simulink model "Octocopter2D_04StatesLin"  (R2020b)
settings: Solver=VariableStepAuto  StartTime=0.0  StopTime=20  RelTol=1e-3
undefined symbols (not defined in the file): A, ACmp, B1, B2, BCmp, C2, CCmp, D21, DCmp, K, xInit
settings Model: Creator=jeremie  LastModifiedBy=jeremie
settings DebuggingCC: ArithmeticOperatorsInVariantConditions=warning
settings SFSimCC: SimUseLocalCustomCode=off  CustomCodeUndefinedFunction=UseInterfaceOnly
settings RTWCC: RTWUseLocalCustomCode=off

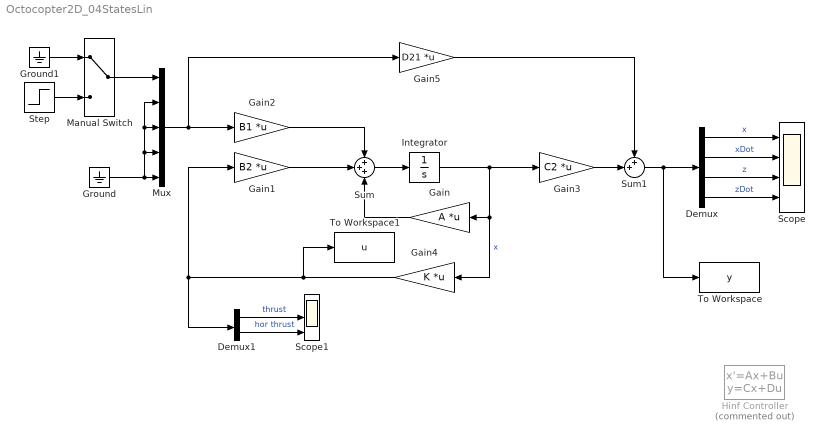
== system Octocopter2D_04StatesLin ==
  Demux : Demux
  Demux1 : Demux  Outputs=2
  Gain : Gain  Gain=A  Multiplication=Matrix(K*u)
  Gain1 : Gain  Gain=B2  Multiplication=Matrix(K*u)
  Gain2 : Gain  Gain=B1  Multiplication=Matrix(K*u)
  Gain3 : Gain  Gain=C2  Multiplication=Matrix(K*u)
  Gain4 : Gain  Gain=K  Multiplication=Matrix(K*u)
  Gain5 : Gain  Gain=D21  Multiplication=Matrix(K*u)
  Ground : Ground
  Ground1 : Ground
  Hinf Controller : StateSpace  Commented=on  A=ACmp  B=BCmp  C=CCmp  D=DCmp  InitialCondition=0
  Integrator : Integrator  InitialCondition=xInit
  Manual Switch : ManualSwitch
  Mux : Mux  Inputs=5
  Scope : Scope  NumInputPorts=4
  Scope1 : Scope  NumInputPorts=3
  Step : Step  Time=10  SampleTime=0
  Sum : Sum  Inputs=+++
  Sum1 : Sum  Inputs=++|
  To Workspace : ToWorkspace  VariableName=y  SampleTime=-1
  To Workspace1 : ToWorkspace  VariableName=u  SampleTime=-1
  wires:
  Gain/1 -> Sum/3
  Integrator/1 -> Gain4/1, Gain/1, Gain3/1  "x"
  Gain1/1 -> Sum/2
  Gain2/1 -> Sum/1
  Sum/1 -> Integrator/1
  Gain3/1 -> Sum1/2
  Gain5/1 -> Sum1/1
  Sum1/1 -> To Workspace/1, Demux/1
  Gain4/1 -> To Workspace1/1, Gain1/1, Demux1/1
  Mux/1 -> Gain2/1, Gain5/1
  Ground/1 -> Mux/2, Mux/3, Mux/4, Mux/5
  Demux/1 -> Scope/1  "x"
  Demux/2 -> Scope/2  "xDot"
  Demux/4 -> Scope/4  "zDot"
  Step/1 -> Manual Switch/2
  Demux1/1 -> Scope1/2  "thrust"
  Demux1/2 -> Scope1/3  "hor thrust"
  Manual Switch/1 -> Mux/1
  Ground1/1 -> Manual Switch/1
  Demux/3 -> Scope/3  "z"
